simulink model "frank"  (R2023b)
settings: Solver=VariableStepAuto  StartTime=0.0  StopTime=5  RelTol=1e-3
values from neighbouring files (symbols this model uses):
  qn = [0, pi/4, pi, 0, pi/4, 0]    [OMPro.m]    (also in OMPro_v1.m = [0, -pi/4, 0, 0, pi/4, 0]; OManPro.m = rand(1,6); moron9dof.m = [0.1 0.1 pi/4 pi/4 -pi/4 pi/4 0 pi/4 0]; testing.m = [0 0 0 0 pi/4 pi/4 0 pi/4 0])
undefined symbols (not defined in the file or in its folder): cinertia, coriolis, nofriction, omega, omega_tilde, p560, transl, troty
libraries: roblocks x39, robotmobilelib x2
settings Model: Creator=jehuy  LastModifiedBy=kangwang

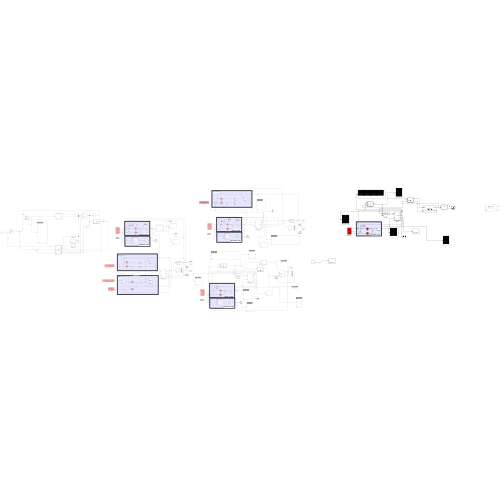
[thumbnail: Simulink's stored preview of the top-level diagram]
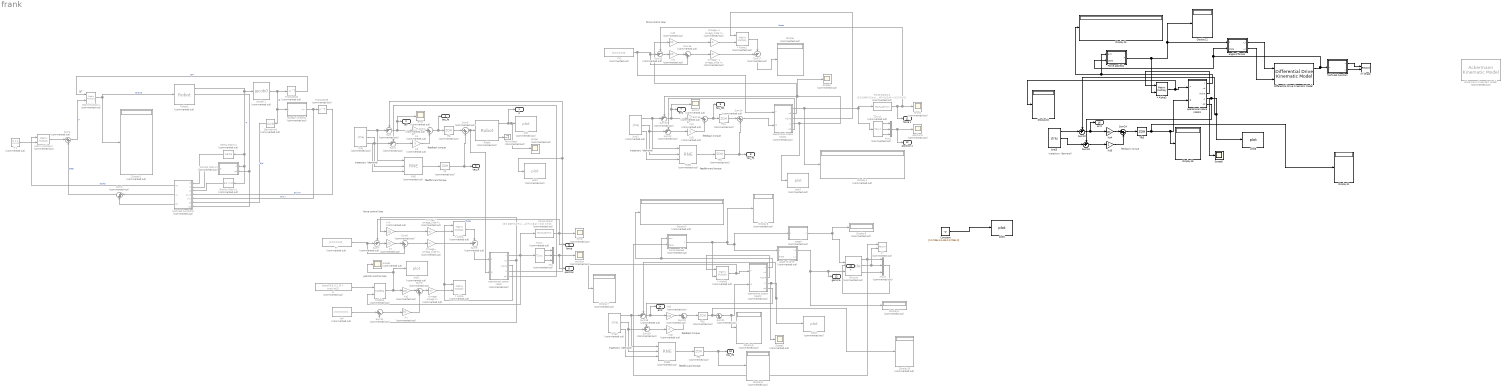
== system frank ==
  note: 0JT
  note: feedforward torque
  note: feedback torque
  note: trajectory
      | (demand)
  note: force control loop
  note: position control loop
  note: feedforward torque
  note: feedback torque
  note: trajectory
      | (demand)
  note: force control loop
  note: feedback torque
  note: trajectory
      | (demand)
  note: feedforward torque
  note: feedback torque
  note: trajectory
      | (demand)
  * Alpha : Product  Commented=on  Multiplication=Matrix(*)
  "* Alpha " : Product  Commented=on  Multiplication=Matrix(*)
  * Alpha1 : Product  Commented=on  Multiplication=Matrix(*)
  * Alpha2 : Product  Commented=on  Multiplication=Matrix(*)
  * Alpha3 : Product  Multiplication=Matrix(*)
  Ackermann Kinematic Model : robotmobilelib/Ackermann Kinematic Model  Commented=on  WheelBase=1  VehicleSpeedRange=[-inf inf]  MaxSteeringAngle=pi/4  InitialState=[0; 0; 0; 0]  SimulateUsing=Interpreted execution
  Bicycle : roblocks/Vehicles/Bicycle  Commented=on  vlim=1  accel=Inf  alim=2  steer_rate=Inf  L=1  x0=[0, 0, 0]
  Constant : Constant  Value=[0 0.7854 3.1416 0 0.7854 0]
  Coriolis Matrix1 : Subsystem  Commented=on  mask{robot=p560}
  Derivative1 : Derivative  Commented=on
  Differential Drive Kinematic Model : robotmobilelib/Differential Drive Kinematic Model  VehicleInputs=Wheel Speeds  WheelRadius=0.05  WheelSpeedRange=[-inf inf]  TrackWidth=0.2  InitialState=[0; 0; 0]  SimulateUsing=Interpreted execution
  Display{,1..10} (11 alike) : Display  Commented=on
  Display{11..13,16,18} (5 alike) : Display
  F'1 : Constant  Commented=on  Value=[0 0 0 0 0 0]'
  F* : Constant  Commented=on  Value=[0 0 0 0 0 0]
  F*2 : Constant  Commented=on  Value=[0 0 0 0 0 0]
  Force applied : MATLAB Function  Commented=on  TreatAsAtomicUnit=on
  Force applied1 : MATLAB Function  TreatAsAtomicUnit=on
  Force sensor : MATLABFcn  Commented=on  MATLABFcn=[0 0 100*(0.2+u(3,4))*(u(3,4)<-0.2) 0 0 0]
  Force sensor1 : MATLABFcn  Commented=on  MATLABFcn=[0 0 100*(0.2+u(3,4))*(u(3,4)<-0.2) 0 0 0]
  Gravity Matrix1 : roblocks/Arm/gravload  Commented=on  robot=p560
  Inertia Matrix1 : roblocks/Arm/inertia  Commented=on  robot=p560
  Kd : Gain  Commented=on  Gain=5  SaturateOnIntegerOverflow=on  OutDataTypeStr=Inherit: Same as input  ParamDataTypeStr=Inherit: Same as input
  Kd1 : Gain  Commented=on  Gain=5  SaturateOnIntegerOverflow=on  OutDataTypeStr=Inherit: Same as input  ParamDataTypeStr=Inherit: Same as input
  Kd2 : Gain  Commented=on  Gain=2  SaturateOnIntegerOverflow=on  OutDataTypeStr=Inherit: Same as input  ParamDataTypeStr=Inherit: Same as input
  Kd3 : Gain  Gain=2  SaturateOnIntegerOverflow=on  OutDataTypeStr=Inherit: Same as input  ParamDataTypeStr=Inherit: Same as input
  Kf : Gain  Commented=on  Gain=20
  Kf1 : Gain  Commented=on  Gain=20
  Kp : Gain  Commented=on  Gain=100  SaturateOnIntegerOverflow=on  OutDataTypeStr=Inherit: Same as input  ParamDataTypeStr=Inherit: Same as input
  Kp1 : Gain  Commented=on  Gain=100
  Kp2 : Gain  Commented=on  Gain=100  SaturateOnIntegerOverflow=on  OutDataTypeStr=Inherit: Same as input  ParamDataTypeStr=Inherit: Same as input
  Kp3 : Gain  Commented=on  Gain=100  SaturateOnIntegerOverflow=on  OutDataTypeStr=Inherit: Same as input  ParamDataTypeStr=Inherit: Same as input
  Kp4 : Gain  Gain=100  SaturateOnIntegerOverflow=on  OutDataTypeStr=Inherit: Same as input  ParamDataTypeStr=Inherit: Same as input
  Kv : Gain  Commented=on  Gain=50
  Kvf : Gain  Commented=on  Gain=20
  Kvf1 : Gain  Commented=on  Gain=20
  MATLAB Function : MATLAB Function  TreatAsAtomicUnit=on
  MATLAB Function2 : MATLAB Function  Commented=on  TreatAsAtomicUnit=on
  Matrix Multiply2 : Product  Commented=on  Multiplication=Matrix(*)
  MatrixMultiply1 : Product  Commented=on  Multiplication=Matrix(*)
  Mux : Mux  Commented=on  Inputs=3
  Mux1 : Mux  Commented=on  Inputs=3
  Mux3 : Mux  Commented=on  Inputs=3
  Omega : Gain  Commented=on  Gain=omega  Multiplication=Matrix(K*u)
  Omega~ : Gain  Commented=on  Gain=omega_tilde  Multiplication=Matrix(K*u)
  "Omega~ " : Gain  Commented=on  Gain=omega_tilde  Multiplication=Matrix(K*u)
  Omega~ 1 : Gain  Commented=on  Gain=omega_tilde  Multiplication=Matrix(K*u)
  Omega~1 : Gain  Commented=on  Gain=omega_tilde  Multiplication=Matrix(K*u)
  RNE : roblocks/Arm/RNE  Commented=on  robot=p560.nofriction()  grav=[0 0 9.81]
  RNE1 : roblocks/Arm/RNE  Commented=on  robot=p560.nofriction()  grav=[0 0 9.81]
  RNE2 : roblocks/Arm/RNE  Commented=on  robot=p560.nofriction()  grav=[0 0 9.81]
  Robot : roblocks/Arm/Robot  Commented=on  robot=p560.nofriction  q0=[0 0 0 0 0 0]
  Robot2 : roblocks/Arm/Robot  Commented=on  robot=p560.nofriction  q0=[0 0 0 0 0 0]
      link override Integrator1: InitialCondition=[0 0 0 0 0 0]
  Scope{,1..3} (4 alike) : Scope  Commented=on
  Scope5 : Scope
  Sum{,1,10,12,18..19} (6 alike) : Sum  Commented=on  Inputs=-+|  InputSameDT=on  SaturateOnIntegerOverflow=on  OutDataTypeStr=Inherit: Same as first input
  Sum11 : Sum  Commented=on  Inputs=|+-
  Sum{4..5,13..14,20..21} (6 alike) : Sum  Commented=on  Inputs=|++  InputSameDT=on  SaturateOnIntegerOverflow=on  OutDataTypeStr=Inherit: Same as first input
  Sum15 : Sum  Commented=on  Inputs=-+|
  Sum{2..3,6,8,16} (5 alike) : Sum  Commented=on  Inputs=|++
  Sum17 : Sum  Commented=on  Inputs=+-|
  Sum22 : Sum  Inputs=-+|  InputSameDT=on  SaturateOnIntegerOverflow=on  OutDataTypeStr=Inherit: Same as first input
  Sum23 : Sum  Inputs=-+|  InputSameDT=on  SaturateOnIntegerOverflow=on  OutDataTypeStr=Inherit: Same as first input
  Sum24 : Sum  Inputs=|++  InputSameDT=on  SaturateOnIntegerOverflow=on  OutDataTypeStr=Inherit: Same as first input
  Sum7 : Sum  Commented=on  Inputs=-+|
  Sum9 : Sum  Commented=on  Inputs=+-|
  T2xyz : roblocks/Toolbox/T2xyz  Commented=on
  T2xyz1 : roblocks/Toolbox/T2xyz  Commented=on
  Terminator : Terminator  Commented=on
  Tfb : ZeroOrderHold  Commented=on  SampleTime=0.002
  Tfb1 : ZeroOrderHold  Commented=on  SampleTime=0.002
  Tfb2 : ZeroOrderHold  Commented=on  SampleTime=0.002
  Tfb3 : ZeroOrderHold  SampleTime=0.002
  Tff : ZeroOrderHold  Commented=on  SampleTime=0.05
  Tff1 : ZeroOrderHold  Commented=on  SampleTime=0.05
  Tff2 : ZeroOrderHold  Commented=on  SampleTime=0.05
  Transpose2 : Math  Commented=on  Operator=transpose
  Transpose3 : Math  Commented=on  Operator=transpose
  XY : Record  Commented=on  FileSettingsInternal="{\"entries\":[{\"content\":{\"excelSettings\":{\"content\":{},\"type\":\"Streamout.ExcelSettings\"}},\"type\":\"Streamout.FileSettingStorage\",\"uuid\":\"\"}],\"packageUris\":[\"http:\\/\\/schema.mathworks.com\\/mf0\\/streamout_blocks\\/R2020a\"],\"version\":\"1.0\"}"  Layout=[1 1]  SignalsInternal="{\"entries\":[{\"content\":{\"signals\":[{\"content\":{\"blockPath\":[],\"dimensions\":[1],\"domain\":\"\",\"lineColor\":\"#fe330a\",\"plots\":[1],\"port\":1,\"signalID\":34,\"signalName\":\"Bicycle:1\"},\"type\":\"RecordBlkView.Signal\",\"uuid\":\"\"},{\"content\":{\"blockPath\":[],\"dimensions\":[1],\"domain\":\"\",\"lineColor\":\"#22b573\",\"plots\":[1],\"port\":2,\"signalID\":37,\"signalName\":\"Bicycle:2\"},\"type\":\"RecordBlkView.Signal\",\"uuid\":\"\"}]},\"type\":\"RecordBlkView.InputSignals\",\"uuid\":\"\"}],\"packageUris\":[\"http:\\/\\/schema.mathworks.com\\/mf0\\/streamout_blocks\\/R2020a\"],\"version\":\"1.0\"}"  VisualizationBindings="{\"xyplotplugin\":{\"info\":[{\"series\":[{\"bindingParametersList\":[{\"parameter\":\"X-Axis\",\"signalID\":34,\"signalName\":\"Bicycle:1\"},{\"parameter\":\"Y-Axis\",\"signalID\":37,\"signalName\":\"Bicycle:2\"}],\"seriesID\":63162}],\"subplotID\":1}]}}"  CompatibilityTag=XY  st=-1
  XY Graph : Record  FileSettingsInternal="{\"entries\":[{\"content\":{\"excelSettings\":{\"content\":{},\"type\":\"Streamout.ExcelSettings\"}},\"type\":\"Streamout.FileSettingStorage\",\"uuid\":\"\"}],\"packageUris\":[\"http:\\/\\/schema.mathworks.com\\/mf0\\/streamout_blocks\\/R2020a\"],\"version\":\"1.0\"}"  Layout=[1 1]  SignalsInternal="{\"entries\":[{\"content\":{\"signals\":[{\"content\":{\"blockPath\":[],\"dimensions\":[1],\"domain\":\"\",\"lineColor\":\"#a2142f\",\"plots\":[1],\"port\":1,\"sid\":[\"\"],\"signalID\":50,\"signalName\":\"MATLAB Function:1\"},\"type\":\"RecordBlkView.Signal\",\"uuid\":\"\"},{\"content\":{\"blockPath\":[],\"dimensions\":[1],\"domain\":\"\",\"lineColor\":\"#139fff\",\"plots\":[1],\"port\":2,\"sid\":[\"\"],\"signalID\":54,\"signalName\":\"MATLAB Function:2\"},\"type\":\"RecordBlkView.Signal\",\"uuid\":\"\"}]},\"type\":\"RecordBlkView.InputSignals\",\"uuid\":\"\"}],\"packageUris\":[\"http:\\/\\/schema.mathworks.com\\/mf0\\/streamout_blocks\\/R2020a\"],\"version\":\"1.0\"}"  VisualizationBindings="{\"xyplotplugin\":{\"info\":[{\"series\":[{\"bindingParametersList\":[{\"parameter\":\"X-Axis\",\"signalID\":50,\"signalName\":\"MATLAB Function:1\"},{\"parameter\":\"Y-Axis\",\"signalID\":54,\"signalName\":\"MATLAB Function:2\"}],\"seriesID\":12818}],\"subplotID\":1}]}}"  CompatibilityTag=XY
  angle of force : MATLAB Function  Commented=on  TreatAsAtomicUnit=on
  angle of force1 : MATLAB Function  TreatAsAtomicUnit=on
  error : Scope  Commented=on
  error1 : Scope  Commented=on
  force : Scope  Commented=on
  force1 : Scope  Commented=on
  jacob0 1 : roblocks/Arm/jacob0   Commented=on  robot=p560
  jtraj : roblocks/Toolbox/jtraj  Commented=on  q0=[0 0 0 0 0 0]  qf=[pi/4 pi/2 -pi/2 0 0 0]  tmax=5  ts=0.02
  jtraj1 : roblocks/Toolbox/jtraj  Commented=on  q0=[0 0 0 0 0 0]  qf=[pi/4 pi/2 -pi/2 0 0 0]  tmax=5  ts=0.02
  jtraj2 : roblocks/Toolbox/jtraj  Commented=on  q0=[0 0.7854 3.1416 0 0.7854 0]  qf=[0 0.7854 3.1416 0 0.7854 0]  tmax=5  ts=0.02
  jtraj3 : roblocks/Toolbox/jtraj  q0=[0 0.7854 3.1416 0 0.7854 0]  qf=[0 0.7854 3.1416 0 0.7854 0]  tmax=5  ts=0.02
  operational space robot : Subsystem  Commented=on  mask{robot=nofriction(p560), q0=qn}
      mask prompts: q0 "Initial joint angles"
  operational space robot1 : Subsystem  Commented=on  mask{robot=nofriction(p560), q0=qn}
      mask prompts: q0 "Initial joint angles"
  operational space robot2 : Subsystem  Commented=on  mask{robot=nofriction(p560), q0=qn}
      mask prompts: q0 "Initial joint angles"
  operational space robot3 : Subsystem  mask{robot=nofriction(p560), q0=qn}
      mask prompts: q0 "Initial joint angles"
  plot{,2..4} (4 alike) : roblocks/Arm/plot  Commented=on  robot=p560  fps=10  holdplot=on
  plot1 : roblocks/Arm/plot  Commented=on  robot=p560  fps=25  holdplot=on
  plot5 : roblocks/Arm/plot  robot=p560  fps=10  holdplot=on
  plot6 : roblocks/Arm/plot  robot=p560  fps=10  holdplot=on
  position : Scope  Commented=on
  position1 : Scope  Commented=on
  psuedo-inverse1 : MATLAB Function  Commented=on  TreatAsAtomicUnit=on
  speed : MATLAB Function  Commented=on  TreatAsAtomicUnit=on
  tr2delta : roblocks/Toolbox/tr2delta  Commented=on
  x* : Constant  Commented=on  Value=transl(0.8, 0.2, 0) * troty(pi/2)
  xd* : Constant  Commented=on  Value=[0 0 0 0 0 0]
  q : Outport
  err : Outport  Port=2
  tau_ff : Outport  Port=3
  tau_fb : Outport  Port=4
  "position " : Outport  Port=5
  "force " : Outport  Port=6
  err1 : Outport  Port=7
  tau_ff1 : Outport  Port=8
  tau_fb1 : Outport  Port=9
  position 1 : Outport  Port=10
  force 1 : Outport  Port=11
  x : Outport  Port=12
  gamma : Outport  Port=13
  err2 : Outport  Port=14
  tau_ff2 : Outport  Port=15
  err3 : Outport  Port=16
  wires:
  MatrixMultiply1/1 -> Robot2/1, Display1/1  "torque"
  MATLAB Function2/2(Vx) -> Sum3/1
  Matrix Multiply2/1 -> Sum2/1
  Inertia Matrix1/1 -> MATLAB Function2/1(M)
  Derivative1/1 -> MATLAB Function2/6(Jd)  "0Jd"
  Sum2/1 -> MatrixMultiply1/2  "F"
  Transpose3/1 -> MATLAB Function2/4(JinvT)  "0JinvT"
  Transpose2/1 -> MatrixMultiply1/1  "0JT"
  Coriolis Matrix1/1(C) -> MATLAB Function2/2(C)
  Sum3/1 -> Sum2/2  "beta"
  F'1/1 -> Matrix Multiply2/2
  MATLAB Function2/3(Gx) -> Sum3/2
  MATLAB Function2/1(Mx) -> Matrix Multiply2/1  "alpha"
  Gravity Matrix1/1 -> MATLAB Function2/3(G)
  psuedo-inverse1/1(Jinv) -> MATLAB Function2/5(Jinv), Transpose3/1  "0Jinv"
  jacob0 1/1 -> psuedo-inverse1/1(J), Derivative1/1, Transpose2/1  "0J"
  Robot2/1 -> Inertia Matrix1/1, Coriolis Matrix1/1(q), Gravity Matrix1/1, jacob0 1/1  "q"
  Robot2/2 -> MATLAB Function2/7(qd), Coriolis Matrix1/2(qd)
  Robot/1 -> Scope/1, plot/1, q/1
  Kd/1 -> Sum4/2
  Kp/1 -> Sum4/1
  Sum/1 -> error/1, err/1, Kp/1
  Sum4/1 -> Tfb/1, tau_fb/1
  jtraj/2 -> Sum1/2, RNE/2
  Tff/1 -> tau_ff/1, Sum5/2
  Sum5/1 -> operational space robot/2(Q), Robot/1
  jtraj/1 -> RNE/1, Sum/2
  jtraj/3 -> RNE/3
  Robot/3 -> Terminator/1
  Sum1/1 -> Kd/1
  RNE/1 -> Tff/1
  Tfb/1 -> Sum5/1
  tr2delta/1 -> Scope1/1, plot1/1, Kp1/1
  operational space robot/3(Alpha) -> * Alpha/1, "* Alpha "/1
  T2xyz/1 -> Mux/1
  Kv/1 -> Sum6/2
  Kp1/1 -> Sum6/1
  operational space robot/2(xd) -> Sum11/2, Kvf/1
  Kf/1 -> Sum8/1
  xd*/1 -> Sum11/1
  Sum6/1 -> Omega/1
  * Alpha/1 -> Sum9/2
  Sum11/1 -> Kv/1
  Mux/1 -> "position "/1, position/1
  F*/1 -> Sum8/2, Sum7/2
  Force sensor/1 -> "force "/1, force/1, Sum7/1  "force"
  operational space robot/1(x) -> Force sensor/1, T2xyz/1, tr2delta/2
  Sum7/1 -> Kf/1
  Kvf/1 -> Omega~/1
  "Omega~ "/1 -> Sum9/1
  Omega/1 -> "* Alpha "/2
  Sum8/1 -> "Omega~ "/1
  x*/1 -> tr2delta/1
  T2xyz/2 -> Mux/2
  T2xyz/3 -> Mux/3
  Omega~/1 -> * Alpha/2
  Sum9/1 -> operational space robot/1(F)
  operational space robot/5(qd) -> Sum1/1
  operational space robot/4(q) -> plot2/1, Sum/1
  RNE1/1 -> Tff1/1
  Tff1/1 -> tau_ff1/1, Sum14/2
  jtraj1/3 -> RNE1/3
  Kd1/1 -> Sum13/2
  Sum14/1 -> operational space robot1/2(Q)
  Sum12/1 -> Kd1/1
  jtraj1/2 -> Sum12/2, RNE1/2
  jtraj1/1 -> RNE1/1, Sum10/2
  Sum10/1 -> error1/1, err1/1, Kp2/1
  Kp2/1 -> Sum13/1
  Sum13/1 -> Tfb1/1, tau_fb1/1
  Tfb1/1 -> Sum14/1
  operational space robot1/4(q) -> plot4/1, Scope2/1, Sum10/1
  operational space robot1/5(qd) -> Sum12/1
  Sum16/1 -> Omega~ 1/1
  * Alpha1/1 -> Sum17/2
  Kf1/1 -> Sum16/1
  Omega~1/1 -> * Alpha1/2
  operational space robot1/3(Alpha) -> * Alpha1/1
  F*2/1 -> operational space robot1/1(F), Sum16/2, Sum15/2
  Kvf1/1 -> Omega~1/1
  Sum15/1 -> Kf1/1
  Omega~ 1/1 -> Sum17/1
  Force sensor1/1 -> force 1/1, force1/1, Sum15/1  "force"
  operational space robot1/2(xd) -> Kvf1/1
  Sum17/1 -> Display/1
  Mux1/1 -> position 1/1, position1/1
  T2xyz1/3 -> Mux1/3
  T2xyz1/1 -> Mux1/1
  T2xyz1/2 -> Mux1/2
  operational space robot1/1(x) -> Display2/1, T2xyz1/1, Force sensor1/1
  operational space robot2/1(x) -> Force applied/1(arm), Display4/1
  Force applied/1(F) -> * Alpha2/2, Display3/1, speed/1(u), angle of force/1(u)
  Bicycle/3 -> Mux3/3
  angle of force/1(v_l) -> Display6/1, gamma/1, Bicycle/2
  Bicycle/1 -> XY/1, Force applied/2(base), Mux3/1
  Bicycle/2 -> Mux3/2, XY/2
  Mux3/1 -> x/1
  speed/1(y) -> Bicycle/1, Display5/1
  Tfb2/1 -> Display10/1, Sum21/1
  Sum21/1 -> Display9/1, operational space robot2/2(Q)
  jtraj2/1 -> RNE2/1, Sum18/2
  Sum18/1 -> err2/1, Kp3/1
  Sum20/1 -> Tfb2/1
  operational space robot2/4(q) -> Scope3/1, Sum18/1, plot3/1
  jtraj2/3 -> RNE2/3
  jtraj2/2 -> Sum19/2, RNE2/2
  RNE2/1 -> Tff2/1
  Kd2/1 -> Sum20/2
  Tff2/1 -> Display8/1, tau_ff2/1
  Kp3/1 -> Sum20/1
  operational space robot2/5(qd) -> Sum19/1
  Sum19/1 -> Kd2/1
  Constant/1 -> plot5/1
  * Alpha2/1 -> Display7/1, operational space robot2/1(F)
  operational space robot2/3(Alpha) -> * Alpha2/1
  operational space robot3/4(q) -> Scope5/1, Sum22/1, plot6/1
  Force applied1/1(F) -> * Alpha3/2, Display12/1, angle of force1/1(F)
  operational space robot3/5(qd) -> Sum23/1
  Sum23/1 -> Kd3/1
  operational space robot3/1(x) -> Force applied1/1(arm), Display13/1
  Sum22/1 -> err3/1, Kp4/1
  Kp4/1 -> Sum24/1
  Sum24/1 -> Tfb3/1
  * Alpha3/1 -> Display16/1, operational space robot3/1(F)
  operational space robot3/3(Alpha) -> * Alpha3/1
  jtraj3/1 -> Sum22/2
  Kd3/1 -> Sum24/2
  jtraj3/2 -> Sum23/2
  Tfb3/1 -> Display18/1, operational space robot3/2(Q), Display11/1
  angle of force1/1(v_l) -> Differential Drive Kinematic Model/1
  angle of force1/2(v_r) -> Differential Drive Kinematic Model/2
  Differential Drive Kinematic Model/1 -> MATLAB Function/1(u), Force applied1/2(state), angle of force1/2(state)
  MATLAB Function/1(x) -> XY Graph/1
  MATLAB Function/2(y) -> XY Graph/2

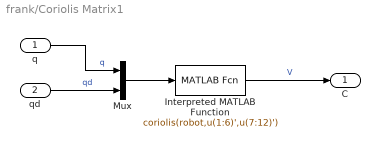
== system frank/Coriolis Matrix1 ==
  q : Inport
  qd : Inport  Port=2
  Interpreted MATLAB Function : MATLABFcn  MATLABFcn=coriolis(robot,u(1:6)',u(7:12)')  Output1D=off
  Mux : Mux  Inputs=2
  C : Outport
  wires:
  Mux/1 -> Interpreted MATLAB Function/1
  q/1 -> Mux/1  "q"
  qd/1 -> Mux/2  "qd"
  Interpreted MATLAB Function/1 -> C/1  "V"

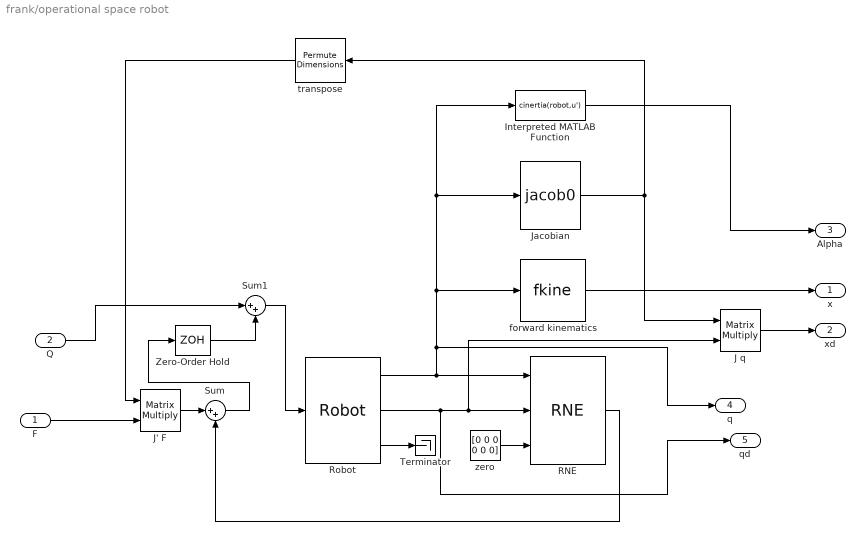
== system frank/operational space robot ==
  F : Inport
  Q : Inport  Port=2
  Interpreted MATLAB Function : MATLABFcn  MATLABFcn=cinertia(robot,u')  OutputDimensions=[6 6]  Output1D=off
  J q : Product  Multiplication=Matrix(*)
  J' F : Product  Multiplication=Matrix(*)
  Jacobian : roblocks/Arm/jacob0   robot=robot
  RNE : roblocks/Arm/RNE  robot=robot  grav=[0 0 9.81]
  Robot : roblocks/Arm/Robot  robot=robot  q0=q0
  Sum : Sum  Inputs=|++
  Sum1 : Sum  Inputs=|++
  Terminator : Terminator
  Zero-Order Hold : ZeroOrderHold  SampleTime=5e-3
  forward kinematics : roblocks/Arm/fkine  robot=robot
  transpose : PermuteDimensions
  zero : Constant  Value=[0 0 0 0 0 0]
  x : Outport
  xd : Outport  Port=2
  Alpha : Outport  Port=3
  q : Outport  Port=4
  qd : Outport  Port=5
  wires:
  Interpreted MATLAB Function/1 -> Alpha/1
  Sum/1 -> Zero-Order Hold/1
  F/1 -> J' F/2
  transpose/1 -> J' F/1
  J' F/1 -> Sum/1
  RNE/1 -> Sum/2
  zero/1 -> RNE/3
  Robot/3 -> Terminator/1
  Robot/2 -> qd/1, RNE/2, J q/2
  Robot/1 -> RNE/1, forward kinematics/1, Interpreted MATLAB Function/1, Jacobian/1, q/1
  forward kinematics/1 -> x/1
  J q/1 -> xd/1
  Jacobian/1 -> transpose/1, J q/1
  Zero-Order Hold/1 -> Sum1/2
  Q/1 -> Sum1/1
  Sum1/1 -> Robot/1

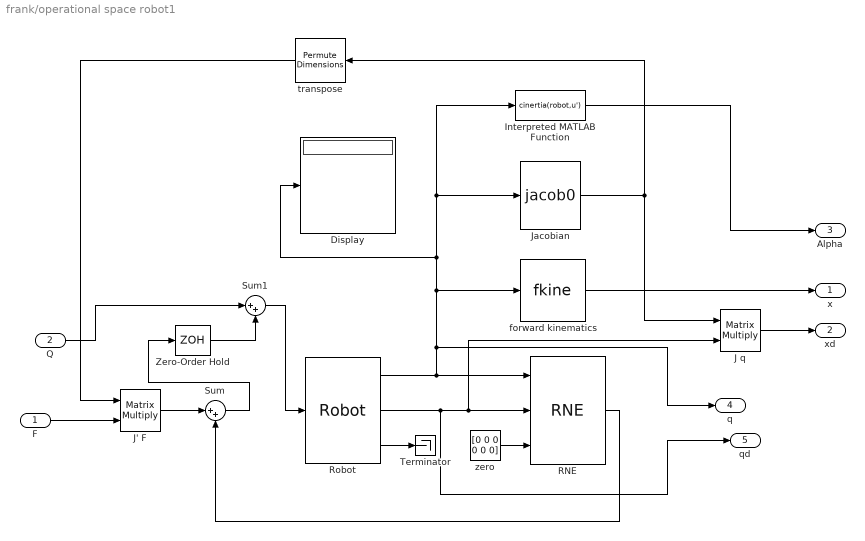
== system frank/operational space robot1 ==
  F : Inport
  Q : Inport  Port=2
  Display : Display
  Interpreted MATLAB Function : MATLABFcn  MATLABFcn=cinertia(robot,u')  OutputDimensions=[6 6]  Output1D=off
  J q : Product  Multiplication=Matrix(*)
  J' F : Product  Multiplication=Matrix(*)
  Jacobian : roblocks/Arm/jacob0   robot=robot
  RNE : roblocks/Arm/RNE  robot=robot  grav=[0 0 9.81]
  Robot : roblocks/Arm/Robot  robot=robot  q0=q0
  Sum : Sum  Inputs=|++
  Sum1 : Sum  Inputs=|++
  Terminator : Terminator
  Zero-Order Hold : ZeroOrderHold  SampleTime=5e-3
  forward kinematics : roblocks/Arm/fkine  robot=robot
  transpose : PermuteDimensions
  zero : Constant  Value=[0 0 0 0 0 0]
  x : Outport
  xd : Outport  Port=2
  Alpha : Outport  Port=3
  q : Outport  Port=4
  qd : Outport  Port=5
  wires:
  Interpreted MATLAB Function/1 -> Alpha/1
  Sum/1 -> Zero-Order Hold/1
  F/1 -> J' F/2
  transpose/1 -> J' F/1
  J' F/1 -> Sum/1
  RNE/1 -> Sum/2
  zero/1 -> RNE/3
  Robot/3 -> Terminator/1
  Robot/2 -> qd/1, RNE/2, J q/2
  Robot/1 -> RNE/1, forward kinematics/1, Interpreted MATLAB Function/1, Jacobian/1, Display/1, q/1
  forward kinematics/1 -> x/1
  J q/1 -> xd/1
  Jacobian/1 -> transpose/1, J q/1
  Q/1 -> Sum1/1
  Sum1/1 -> Robot/1
  Zero-Order Hold/1 -> Sum1/2

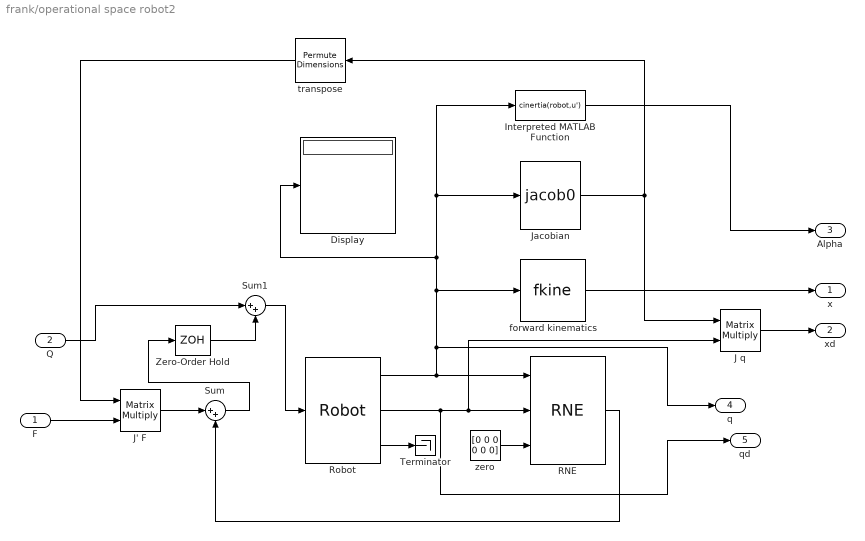
== system frank/operational space robot2 ==
  F : Inport
  Q : Inport  Port=2
  Display : Display
  Interpreted MATLAB Function : MATLABFcn  MATLABFcn=cinertia(robot,u')  OutputDimensions=[6 6]  Output1D=off
  J q : Product  Multiplication=Matrix(*)
  J' F : Product  Multiplication=Matrix(*)
  Jacobian : roblocks/Arm/jacob0   robot=robot
  RNE : roblocks/Arm/RNE  robot=robot  grav=[0 0 9.81]
  Robot : roblocks/Arm/Robot  robot=robot  q0=q0
  Sum : Sum  Inputs=|++
  Sum1 : Sum  Inputs=|++
  Terminator : Terminator
  Zero-Order Hold : ZeroOrderHold  SampleTime=5e-3
  forward kinematics : roblocks/Arm/fkine  robot=robot
  transpose : PermuteDimensions
  zero : Constant  Value=[0 0 0 0 0 0]
  x : Outport
  xd : Outport  Port=2
  Alpha : Outport  Port=3
  q : Outport  Port=4
  qd : Outport  Port=5
  wires:
  Interpreted MATLAB Function/1 -> Alpha/1
  Sum/1 -> Zero-Order Hold/1
  F/1 -> J' F/2
  transpose/1 -> J' F/1
  J' F/1 -> Sum/1
  RNE/1 -> Sum/2
  zero/1 -> RNE/3
  Robot/3 -> Terminator/1
  Robot/2 -> qd/1, RNE/2, J q/2
  Robot/1 -> RNE/1, forward kinematics/1, Interpreted MATLAB Function/1, Jacobian/1, Display/1, q/1
  forward kinematics/1 -> x/1
  J q/1 -> xd/1
  Jacobian/1 -> transpose/1, J q/1
  Q/1 -> Sum1/1
  Sum1/1 -> Robot/1
  Zero-Order Hold/1 -> Sum1/2

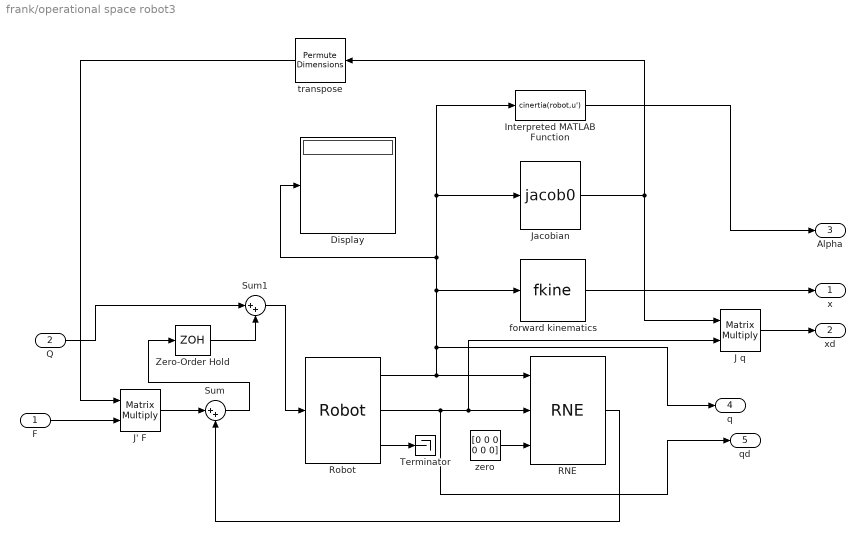
== system frank/operational space robot3 ==
  F : Inport
  Q : Inport  Port=2
  Display : Display
  Interpreted MATLAB Function : MATLABFcn  MATLABFcn=cinertia(robot,u')  OutputDimensions=[6 6]  Output1D=off
  J q : Product  Multiplication=Matrix(*)
  J' F : Product  Multiplication=Matrix(*)
  Jacobian : roblocks/Arm/jacob0   robot=robot
  RNE : roblocks/Arm/RNE  robot=robot  grav=[0 0 9.81]
  Robot : roblocks/Arm/Robot  robot=robot  q0=q0
  Sum : Sum  Inputs=|++
  Sum1 : Sum  Inputs=|++
  Terminator : Terminator
  Zero-Order Hold : ZeroOrderHold  SampleTime=5e-3
  forward kinematics : roblocks/Arm/fkine  robot=robot
  transpose : PermuteDimensions
  zero : Constant  Value=[0 0 0 0 0 0]
  x : Outport
  xd : Outport  Port=2
  Alpha : Outport  Port=3
  q : Outport  Port=4
  qd : Outport  Port=5
  wires:
  Interpreted MATLAB Function/1 -> Alpha/1
  Sum/1 -> Zero-Order Hold/1
  F/1 -> J' F/2
  transpose/1 -> J' F/1
  J' F/1 -> Sum/1
  RNE/1 -> Sum/2
  zero/1 -> RNE/3
  Robot/3 -> Terminator/1
  Robot/2 -> qd/1, RNE/2, J q/2
  Robot/1 -> RNE/1, forward kinematics/1, Interpreted MATLAB Function/1, Jacobian/1, Display/1, q/1
  forward kinematics/1 -> x/1
  J q/1 -> xd/1
  Jacobian/1 -> transpose/1, J q/1
  Q/1 -> Sum1/1
  Sum1/1 -> Robot/1
  Zero-Order Hold/1 -> Sum1/2

== matlab function frank/Force applied ==
  data: arm input; F output; base input
function F = fcn(arm,base)
x_arm = arm(1,4);
x_base = base;
x = x_base+x_arm;
F = [0 0 0 0 0 0].';
if x < 1.8 
    F = [5 0 0 0 0 0].';
end

== matlab function frank/MATLAB Function2 ==
  data: M input; Mx output; C input; G input; JinvT input; Jinv input; Jd input; qd input; Vx output; Gx output
function [Mx,Vx,Gx]= fcn(M,C,G,JinvT,Jinv,Jd,qd)

V=C*qd;

Mx=JinvT*M*Jinv;
Gx=JinvT*G';
Vx=JinvT*(V-M*Jinv*Jd*qd);

== matlab function frank/angle of force ==
  data: u input; v_l output; v_r output; theta input
function [v_l, v_r]= fcn(u, theta)
Fx = F(1);
Fy = F(2);

theta = atan2(Fy, Fx);         % Direction of force
speed = norm([Fx, Fy]);        % Magnitude of force

% Motion command
v = speed;  % linear speed
w = 0;      % no angular velocity for now

% Robot parameters
r = 0.05;   % wheel radius (m)
L = 0.2;    % distance between wheels (m)

% Convert to wheel speeds
v_l = (2*v - w*L)/(2*r);
v_r = (2*v + w*L)/(2*r);

== matlab function frank/psuedo-inverse1 ==
  data: J input; Jinv output
function Jinv = fcn(J)

Jinv = pinv(J);

== matlab function frank/speed ==
  data: u input; y output
function y = fcn(u)

y = norm(u);

== matlab function frank/Force applied1 ==
  data: arm input; F output; state input
function F = fcn(arm,state)
x_arm = arm(1,4);
x_base = state(1);
x = x_base+x_arm;
F = [0 0 0 0 0 0].';
if x < 1.8 
    F = [5 0 0 0 0 0].';
end

== matlab function frank/angle of force1 ==
  data: F input; v_l output; v_r output; state input
function [v_l, v_r]= fcn(F, state)
current_heading = state(3);           
k_theta = 2.0;                    

r = 0.05;                         
L = 0.2;                          

Fx = F(1);
Fy = F(2);
force_angle = atan2(Fy, Fx);
speed = norm([Fx, Fy]);

error_theta = wrapToPi(force_angle - current_heading);
w = k_theta * error_theta;

v = speed;  

v_l = (2*v - w*L)/(2*r);
v_r = (2*v + w*L)/(2*r);

== matlab function frank/MATLAB Function ==
  data: x output; u input; y output
function [x,y]= fcn(u)

x = u(1);
y = u(2);
